simulink model "power_48pulsegtoconverter"  (R2013a)
settings: Solver=FixedStepDiscrete  SolverMode=SingleTasking  StartTime=0.0  StopTime=0.05  RelTol=1e-3
libraries: powerlib x17, powerlib_extras x1
(part 1 of 2)
Description:
  | Copyright 2008-2013 The MathWorks, Inc.
settings Model: ExtModeTrigMode=oneshot  ExtModeArmWhenConnect=off  ExtModeAutoUpdateStatusClock=off  Creator=MathWorks  LastModifiedBy=nau03113
settings DataIOCC: LimitDataPoints=off  SignalLoggingSaveFormat=ModelDataLogs  SaveOutput=off  SaveTime=off  SignalLoggingName=sigsOut
settings OptimizationCC: BlockReduction=off  BooleanDataType=off  ExpressionDepthLimit=2147483647  InitFltsAndDblsToZero=on
settings DebuggingCC: SaveWithParameterizedLinksMsg=none  CheckExecutionContextPreStartOutputMsg=on  CheckExecutionContextRuntimeOutputMsg=on  SignalResolutionControl=TryResolveAllWithWarning  SolverPrmCheckMsg=none  MultiTaskDSMMsg=warning  MultiTaskCondExecSysMsg=none  FcnCallInpInsideContextMsg=UseLocalSettings
settings HardwareCC: TargetUnknown=on
settings RTWCC: IncludeERTFirstTime=on
settings GRTTargetCC: TargetFcnLib=ansi_tfl_tmw.mat  CombineOutputUpdateFcns=off  GRTInterface=on

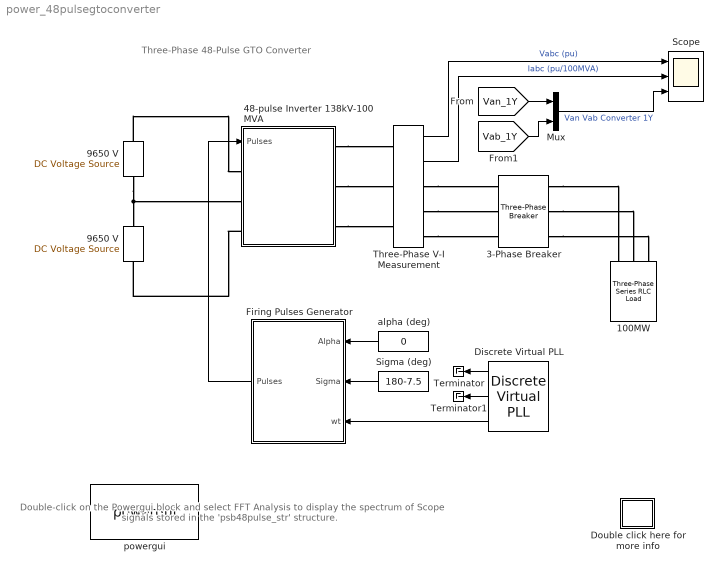
== system power_48pulsegtoconverter ==
  note: Three-Phase 48-Pulse GTO Converter
  note: Double-click on the Powergui block and
      | select FFT Analysis to display the
      | spectrum of Scope signals stored in the
      | 'psb48pulse_str' structure.
  100MW : powerlib/Elements/Three-Phase Series RLC Load  LConnTagsString=A|B|C  Configuration=Y (grounded)  NominalVoltage=138e3  NominalFrequency=60  ActivePower=100e6  InductivePower=0  CapacitivePower=0  Measurements=None  LoadType=constant Z
  3-Phase Breaker : powerlib/Elements/Three-Phase Breaker  InitialState=open  SwitchA=on  SwitchB=on  SwitchC=on  SwitchTimes=[0.025]  External=off  BreakerResistance=0.001  SnubberResistance=1e6  SnubberCapacitance=inf  Measurements=None
      settings: AttributesFormatString=\n
  48-pulse Inverter 138kV-100 MVA : Subsystem
  "9650 V " : powerlib/Electrical Sources/DC Voltage Source  Description=source block  Amplitude=9650  Measurements=None
      settings: AttributesFormatString=\n
  "9650 V  " : powerlib/Electrical Sources/DC Voltage Source  Description=source block  Amplitude=9650  Measurements=None
      settings: AttributesFormatString=\n
  Discrete Virtual PLL : powerlib_extras/Discrete  Control Blocks/Discrete Virtual PLL  Freq=60  Phase=0  Ts=5e-6
  Double click here for more info : Subsystem
      settings: OpenFcn=showdemo(bdroot(gcb))
      mask Display: disp('?')
  Firing Pulses Generator : Subsystem
  Mux : Mux  Inputs=2
  Scope : Scope  NumInputPorts=3
      settings: TimeRange=0.05  YMin=-2~-1~-20000  YMax=2~1~20000  SaveName=psb48pulse_str  SampleInput=on
  Sigma (deg) : Constant  Value=180-7.5
  Terminator : Terminator
  Terminator1 : Terminator
  Three-Phase V-I Measurement : powerlib/Measurements/Three-Phase V-I Measurement  VoltageMeasurement=phase-to-ground  SetLabelV=off  LabelV=V1  Vpu=on  VpuLL=off  CurrentMeasurement=yes  SetLabelI=off  LabelI=I1  Ipu=on  Pbase=100e6  Vbase=138e3  OutputType=Magnitude  PhasorSimulation=off  PSBequivalent=0
  alpha (deg) : Constant  Value=0  VectorParams1D=off
  powergui : powerlib/powergui  Priority=2  SimulationMode=Discrete  SolverType=Tustin  SampleTime=5e-6  frequency=60  SPID=off  DisableSnubberDevices=off  DisableRonSwitches=off  DisableVfSwitches=off  SwTol=0  Interpol=off  DisplayEquations=off  frequencyindice=1  Pbase=100e6  ErrMax=1e-4  Iterations=50  UnitsV=kV  UnitsW=MW  FunctionMessages=off  echomessages=off  HookPort=off  EnableUseOfTLC=off  x0status=blocks  RestoreLinks=warning  ResistiveCurrentMeasurement=off  Frange=logspace(0,3,50)  Ylog=off  Xlog=off  ShowGrid=off  save=off  variable=ZData  structure=psb48pulse_str  ZoomFFT=on  StartTime=0.025-1/60  cycles=1  DisplayStyle=off  fundamental=60  FreqAxis=on  MaxFrequency=4000  frequencyindicesteady=1  RmsSteady=1  display=off  Ts=0  methode=off
  wires:
  Sigma (deg)/1 -> Firing Pulses Generator/2(Sigma)
  Discrete Virtual PLL/1 -> Terminator/1
  Discrete Virtual PLL/2 -> Terminator1/1
  Firing Pulses Generator/1(Pulses) -> 48-pulse Inverter 138kV-100 MVA/1(Pulses)
  Discrete Virtual PLL/3 -> Firing Pulses Generator/3(wt)
  alpha (deg)/1 -> Firing Pulses Generator/1(Alpha)
  [Van_1Y] -> Mux/1
  [Vab_1Y] -> Mux/2
  Three-Phase V-I Measurement/1 -> Scope/1  "Vabc (pu)"
  Mux/1 -> Scope/3  "Van Vab Converter 1Y"
  Three-Phase V-I Measurement/2 -> Scope/2  "Iabc (pu/100MVA)"
  connections:
  3-Phase Breaker/RConn1 -- 100MW/LConn1
  3-Phase Breaker/RConn2 -- 100MW/LConn2
  3-Phase Breaker/RConn3 -- 100MW/LConn3
  "9650 V  "/LConn1 -- "9650 V "/RConn1 -- 48-pulse Inverter 138kV-100 MVA/LConn2
  48-pulse Inverter 138kV-100 MVA/RConn1 -- Three-Phase V-I Measurement/LConn1
  48-pulse Inverter 138kV-100 MVA/RConn2 -- Three-Phase V-I Measurement/LConn2
  48-pulse Inverter 138kV-100 MVA/RConn3 -- Three-Phase V-I Measurement/LConn3
  Three-Phase V-I Measurement/RConn1 -- 3-Phase Breaker/LConn1
  Three-Phase V-I Measurement/RConn2 -- 3-Phase Breaker/LConn2
  Three-Phase V-I Measurement/RConn3 -- 3-Phase Breaker/LConn3
  "9650 V  "/RConn1 -- 48-pulse Inverter 138kV-100 MVA/LConn1
  48-pulse Inverter 138kV-100 MVA/LConn3 -- "9650 V "/LConn1

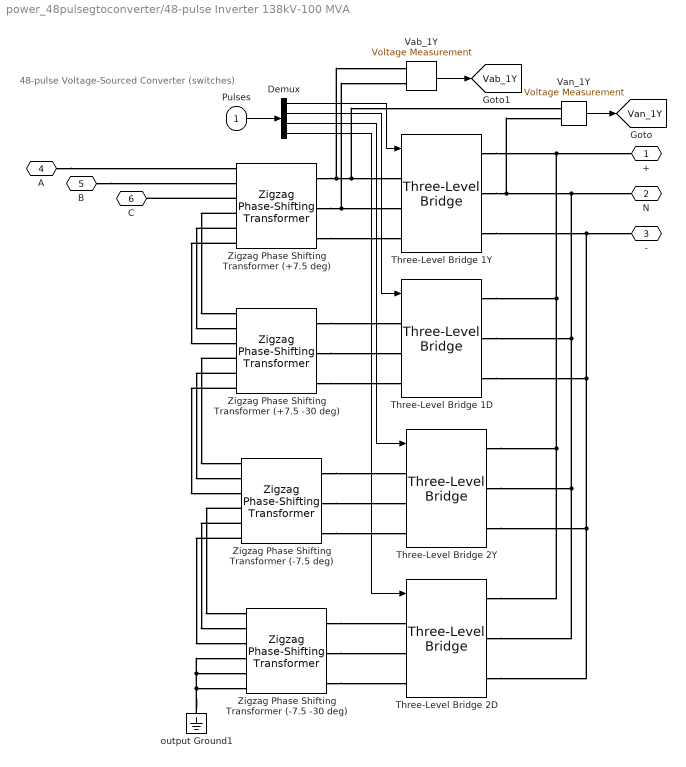
== system power_48pulsegtoconverter/48-pulse Inverter 138kV-100 MVA ==
  note: 48-pulse Voltage-Sourced Converter
      | (switches)
  Pulses : Inport  PortDimensions=48
  Demux : Demux  Outputs=[12 12 12 12]
  Three-Level Bridge 1D : powerlib/Power Electronics/Three-Level Bridge  Arms=3  SnubberResistance=1e6  SbubberCapacitance=inf  Device=Ideal Switches  Ron=1e-4  ForwardVoltages="[  0  0  ]"  Measurements=None
  Three-Level Bridge 1Y : powerlib/Power Electronics/Three-Level Bridge  Arms=3  SnubberResistance=1e6  SbubberCapacitance=inf  Device=Ideal Switches  Ron=1e-4  ForwardVoltages="[  0  0  ]"  Measurements=None
  Three-Level Bridge 2D : powerlib/Power Electronics/Three-Level Bridge  Arms=3  SnubberResistance=1e6  SbubberCapacitance=inf  Device=Ideal Switches  Ron=1e-4  ForwardVoltages="[  0  0  ]"  Measurements=None
  Three-Level Bridge 2Y : powerlib/Power Electronics/Three-Level Bridge  Arms=3  SnubberResistance=1e6  SbubberCapacitance=inf  Device=Ideal Switches  Ron=1e-4  ForwardVoltages="[  0  0  ]"  Measurements=None
  Vab_1Y : powerlib/Measurements/Voltage Measurement  Tag=PoWeRsYsTeMmEaSuReMeNt  PhasorSimulation=off  OutputType=Magnitude  PSBequivalent=0
  Van_1Y : powerlib/Measurements/Voltage Measurement  Tag=PoWeRsYsTeMmEaSuReMeNt  PhasorSimulation=off  OutputType=Magnitude  PSBequivalent=0
  Zigzag Phase Shifting Transformer (+7.5 -30 deg) : powerlib/Elements/Zigzag Phase-Shifting Transformer  SecondaryConnection=Delta D1(-30 deg.)  UNITS=pu  NominalPower=[ 25e6 60]  PrimaryVoltage=138e3/4  SecondaryVoltage="[ 15e3  +7.5]"  Winding1=[ 0.00125 0.05 ]  Winding2=[ 0.00125 0.05 ]  Winding3=[ 0.00125 0.05 ]  SetSaturation=off  RmLm=[ 500 500 ]  Rm=500  Saturation="[ 0,0  ;  0.005,1.2  ;  1.0,1.4 ]"  SetInitialFlux=off  Measurements=Fluxes and magnetization currents (Imag)  InitialFluxes=[0,0,0]  MoreParameters=off  BreakLoop=off  DataType=off
      settings: AttributesFormatString=\n
  Zigzag Phase Shifting Transformer (+7.5 deg) : powerlib/Elements/Zigzag Phase-Shifting Transformer  SecondaryConnection=Y  UNITS=pu  NominalPower=[ 25e6 60]  PrimaryVoltage=138e3/4  SecondaryVoltage="[ 15e3  +7.5]"  Winding1=[ 0.00125 0.05 ]  Winding2=[ 0.00125 0.05 ]  Winding3=[ 0.00125 0.05 ]  SetSaturation=off  RmLm=[ 500 500 ]  Rm=500  Saturation="[ 0,0  ;  0.005,1.2  ;  1.0,1.4 ]"  SetInitialFlux=off  Measurements=Fluxes and excitation currents (Imag + IRm)  InitialFluxes=[0,0,0]  MoreParameters=off  BreakLoop=off  DataType=off
      settings: AttributesFormatString=\n
  Zigzag Phase Shifting Transformer (-7.5 -30 deg) : powerlib/Elements/Zigzag Phase-Shifting Transformer  SecondaryConnection=Delta D1(-30 deg.)  UNITS=pu  NominalPower=[ 25e6 60]  PrimaryVoltage=138e3/4  SecondaryVoltage="[ 15e3  -7.5]"  Winding1=[ 0.00125 0.05 ]  Winding2=[ 0.00125 0.05 ]  Winding3=[ 0.00125 0.05 ]  SetSaturation=off  RmLm=[ 500 500 ]  Rm=500  Saturation="[ 0,0  ;  0.005,1.2  ;  1.0,1.4 ]"  SetInitialFlux=off  Measurements=None  InitialFluxes=[0,0,0]  MoreParameters=off  BreakLoop=off  DataType=off
      settings: AttributesFormatString=\n
  Zigzag Phase Shifting Transformer (-7.5 deg) : powerlib/Elements/Zigzag Phase-Shifting Transformer  SecondaryConnection=Y  UNITS=pu  NominalPower=[ 25e6 60]  PrimaryVoltage=138e3/4  SecondaryVoltage="[ 15e3  -7.5]"  Winding1=[ 0.00125 0.05 ]  Winding2=[ 0.00125 0.05 ]  Winding3=[ 0.00125 0.05 ]  SetSaturation=off  RmLm=[ 500 500 ]  Rm=500  Saturation="[ 0,0  ;  0.005,1.2  ;  1.0,1.4 ]"  SetInitialFlux=off  Measurements=None  InitialFluxes=[0,0,0]  MoreParameters=off  BreakLoop=off  DataType=off
      settings: AttributesFormatString=\n
  output Ground1 : powerlib/Elements/Ground  LConnTagsString=a
  + : PMIOPort  Port=1  Side=Left
  N : PMIOPort  Port=2  Side=Left
  - : PMIOPort  Port=3  Side=Left
  A : PMIOPort  Port=4  Side=Right
  B : PMIOPort  Port=5  Side=Right
  C : PMIOPort  Port=6  Side=Right
  tag scope: Vab_1Y=global, Van_1Y=global
  wires:
  Pulses/1 -> Demux/1
  Van_1Y/1 -> [Van_1Y]
  Vab_1Y/1 -> [Vab_1Y]
  Demux/1 -> Three-Level Bridge 1Y/1
  Demux/2 -> Three-Level Bridge 1D/1
  Demux/3 -> Three-Level Bridge 2Y/1
  Demux/4 -> Three-Level Bridge 2D/1
  connections:
  output Ground1/LConn1 -- Zigzag Phase Shifting Transformer (-7.5 -30 deg)/LConn5 -- Zigzag Phase Shifting Transformer (-7.5 -30 deg)/LConn4 -- Zigzag Phase Shifting Transformer (-7.5 -30 deg)/LConn6
  Zigzag Phase Shifting Transformer (+7.5 -30 deg)/RConn1 -- Three-Level Bridge 1D/LConn1
  Zigzag Phase Shifting Transformer (+7.5 -30 deg)/RConn2 -- Three-Level Bridge 1D/LConn2
  Zigzag Phase Shifting Transformer (+7.5 -30 deg)/RConn3 -- Three-Level Bridge 1D/LConn3
  Zigzag Phase Shifting Transformer (-7.5 deg)/RConn1 -- Three-Level Bridge 2Y/LConn1
  Zigzag Phase Shifting Transformer (-7.5 deg)/RConn2 -- Three-Level Bridge 2Y/LConn2
  Zigzag Phase Shifting Transformer (-7.5 deg)/RConn3 -- Three-Level Bridge 2Y/LConn3
  Zigzag Phase Shifting Transformer (-7.5 -30 deg)/RConn1 -- Three-Level Bridge 2D/LConn1
  Zigzag Phase Shifting Transformer (-7.5 -30 deg)/RConn2 -- Three-Level Bridge 2D/LConn2
  Zigzag Phase Shifting Transformer (-7.5 -30 deg)/RConn3 -- Three-Level Bridge 2D/LConn3
  A/RConn1 -- Zigzag Phase Shifting Transformer (+7.5 deg)/LConn1
  B/RConn1 -- Zigzag Phase Shifting Transformer (+7.5 deg)/LConn2
  Zigzag Phase Shifting Transformer (+7.5 deg)/LConn3 -- C/RConn1
  Zigzag Phase Shifting Transformer (+7.5 deg)/RConn2 -- Three-Level Bridge 1Y/LConn2 -- Vab_1Y/LConn2
  Zigzag Phase Shifting Transformer (+7.5 deg)/RConn1 -- Vab_1Y/LConn1 -- Three-Level Bridge 1Y/LConn1 -- Van_1Y/LConn1
  Zigzag Phase Shifting Transformer (+7.5 deg)/RConn3 -- Three-Level Bridge 1Y/LConn3
  Zigzag Phase Shifting Transformer (+7.5 deg)/LConn4 -- Zigzag Phase Shifting Transformer (+7.5 -30 deg)/LConn1
  Zigzag Phase Shifting Transformer (+7.5 deg)/LConn5 -- Zigzag Phase Shifting Transformer (+7.5 -30 deg)/LConn2
  Zigzag Phase Shifting Transformer (+7.5 deg)/LConn6 -- Zigzag Phase Shifting Transformer (+7.5 -30 deg)/LConn3
  Zigzag Phase Shifting Transformer (+7.5 -30 deg)/LConn4 -- Zigzag Phase Shifting Transformer (-7.5 deg)/LConn1
  Zigzag Phase Shifting Transformer (+7.5 -30 deg)/LConn5 -- Zigzag Phase Shifting Transformer (-7.5 deg)/LConn2
  Zigzag Phase Shifting Transformer (+7.5 -30 deg)/LConn6 -- Zigzag Phase Shifting Transformer (-7.5 deg)/LConn3
  Zigzag Phase Shifting Transformer (-7.5 deg)/LConn5 -- Zigzag Phase Shifting Transformer (-7.5 -30 deg)/LConn2
  Three-Level Bridge 1Y/RConn2 -- N/RConn1 -- Three-Level Bridge 1D/RConn2 -- Three-Level Bridge 2D/RConn2 -- Three-Level Bridge 2Y/RConn2 -- Van_1Y/LConn2
  Three-Level Bridge 2D/RConn1 -- Three-Level Bridge 2Y/RConn1 -- Three-Level Bridge 1Y/RConn1 -- +/RConn1 -- Three-Level Bridge 1D/RConn1
  Three-Level Bridge 2D/RConn3 -- Three-Level Bridge 2Y/RConn3 -- Three-Level Bridge 1Y/RConn3 -- -/RConn1 -- Three-Level Bridge 1D/RConn3
  Zigzag Phase Shifting Transformer (-7.5 deg)/LConn4 -- Zigzag Phase Shifting Transformer (-7.5 -30 deg)/LConn1
  Zigzag Phase Shifting Transformer (-7.5 deg)/LConn6 -- Zigzag Phase Shifting Transformer (-7.5 -30 deg)/LConn3

== system power_48pulsegtoconverter/Double click here for more info ==

== system power_48pulsegtoconverter/Firing Pulses Generator ==
  Alpha : Inport  PortDimensions=1
  Sigma : Inport  Port=2  PortDimensions=1
  wt : Inport  Port=3  PortDimensions=1
  Bridge 1D : Subsystem
  "Bridge 1Y " : Subsystem
  Bridge 2D : Subsystem
  Bridge 2Y : Subsystem
  Constant : Constant  Value=[0 -30 -15 -45]*pi/180
  Deg->Rad : Gain  Gain=pi/180  SaturateOnIntegerOverflow=on  OutDataTypeStr=Inherit: Same as input  ParamDataTypeStr=Inherit: Same as input
  "Deg->Rad " : Gain  Gain=pi/180  SaturateOnIntegerOverflow=on  OutDataTypeStr=Inherit: Same as input  ParamDataTypeStr=Inherit: Same as input
  Demux : Demux
  Mux : Mux  Inputs=[12 12 12 12]
  Sum : Sum  SaturateOnIntegerOverflow=on  InputSameDT=on  OutDataTypeStr=Inherit: Same as first input
  Pulses : Outport
  wires:
  Alpha/1 -> Deg->Rad/1
  Constant/1 -> Sum/2
  "Bridge 1Y "/1(Pulses) -> Mux/1
  Mux/1 -> Pulses/1
  Demux/1 -> "Bridge 1Y "/1(wt)
  Sigma/1 -> "Deg->Rad "/1
  Demux/2 -> Bridge 1D/1(wt)
  Demux/3 -> Bridge 2Y/1(wt)
  Demux/4 -> Bridge 2D/1(wt)
  Deg->Rad/1 -> "Bridge 1Y "/2(Alpha), Bridge 2Y/2(Alpha), Bridge 2D/2(Alpha), Bridge 1D/2(Alpha)
  "Deg->Rad "/1 -> "Bridge 1Y "/3(Sigma), Bridge 1D/3(Sigma), Bridge 2Y/3(Sigma), Bridge 2D/3(Sigma)
  Bridge 1D/1(Pulses) -> Mux/2
  Bridge 2Y/1(Pulses) -> Mux/3
  Bridge 2D/1(Pulses) -> Mux/4
  wt/1 -> Sum/1
  Sum/1 -> Demux/1

== system power_48pulsegtoconverter/Firing Pulses Generator/Bridge 1D ==
  wt : Inport  PortDimensions=1
  Alpha : Inport  Port=2  PortDimensions=1
  Sigma : Inport  Port=3  PortDimensions=1
  Constant : Constant  Value=-2*pi/3
  Constant1 : Constant  Value=2*pi/3
  Mux1 : Mux  Inputs=[4 4 4]
  Phase A : Subsystem
  Phase B : Subsystem
  Phase C : Subsystem
  Sum : Sum  SaturateOnIntegerOverflow=on  InputSameDT=on  OutDataTypeStr=Inherit: Same as first input
  Sum1 : Sum  SaturateOnIntegerOverflow=on  InputSameDT=on  OutDataTypeStr=Inherit: Same as first input
  Sum2 : Sum  SaturateOnIntegerOverflow=on  InputSameDT=on  OutDataTypeStr=Inherit: Same as first input
  Pulses : Outport
  wires:
  Constant1/1 -> Sum1/2
  Sigma/1 -> Phase A/2(sigma), Phase C/2(sigma), Phase B/2(sigma)
  Alpha/1 -> Sum2/2
  wt/1 -> Sum2/1
  Sum2/1 -> Phase A/1(wt), Sum/1, Sum1/1
  Mux1/1 -> Pulses/1
  Phase A/1(Pulses) -> Mux1/1
  Constant/1 -> Sum/2
  Sum/1 -> Phase B/1(wt)
  Sum1/1 -> Phase C/1(wt)
  Phase B/1(Pulses) -> Mux1/2
  Phase C/1(Pulses) -> Mux1/3

== system power_48pulsegtoconverter/Firing Pulses Generator/Bridge 1Y  ==
  wt : Inport  PortDimensions=1
  Alpha : Inport  Port=2  PortDimensions=1
  Sigma : Inport  Port=3  PortDimensions=1
  Constant : Constant  Value=-2*pi/3
  Constant1 : Constant  Value=2*pi/3
  Mux1 : Mux  Inputs=[4 4 4]
  Phase A : Subsystem
  Phase B : Subsystem
  Phase C : Subsystem
  Sum : Sum  SaturateOnIntegerOverflow=on  InputSameDT=on  OutDataTypeStr=Inherit: Same as first input
  Sum1 : Sum  SaturateOnIntegerOverflow=on  InputSameDT=on  OutDataTypeStr=Inherit: Same as first input
  Sum2 : Sum  SaturateOnIntegerOverflow=on  InputSameDT=on  OutDataTypeStr=Inherit: Same as first input
  Pulses : Outport
  wires:
  Phase C/1(Pulses) -> Mux1/3
  Phase B/1(Pulses) -> Mux1/2
  Sum1/1 -> Phase C/1(wt)
  Sum/1 -> Phase B/1(wt)
  Constant/1 -> Sum/2
  Phase A/1(Pulses) -> Mux1/1
  Mux1/1 -> Pulses/1
  Sum2/1 -> Sum1/1, Sum/1, Phase A/1(wt)
  wt/1 -> Sum2/1
  Alpha/1 -> Sum2/2
  Sigma/1 -> Phase B/2(sigma), Phase C/2(sigma), Phase A/2(sigma)
  Constant1/1 -> Sum1/2

== system power_48pulsegtoconverter/Firing Pulses Generator/Bridge 2D ==
  wt : Inport  PortDimensions=1
  Alpha : Inport  Port=2  PortDimensions=1
  Sigma : Inport  Port=3  PortDimensions=1
  Constant : Constant  Value=-2*pi/3
  Constant1 : Constant  Value=2*pi/3
  Mux1 : Mux  Inputs=[4 4 4]
  Phase A : Subsystem
  Phase B : Subsystem
  Phase C : Subsystem
  Sum : Sum  SaturateOnIntegerOverflow=on  InputSameDT=on  OutDataTypeStr=Inherit: Same as first input
  Sum1 : Sum  SaturateOnIntegerOverflow=on  InputSameDT=on  OutDataTypeStr=Inherit: Same as first input
  Sum2 : Sum  SaturateOnIntegerOverflow=on  InputSameDT=on  OutDataTypeStr=Inherit: Same as first input
  Pulses : Outport
  wires:
  Constant1/1 -> Sum1/2
  Sigma/1 -> Phase A/2(sigma), Phase C/2(sigma), Phase B/2(sigma)
  Alpha/1 -> Sum2/2
  wt/1 -> Sum2/1
  Sum2/1 -> Phase A/1(wt), Sum/1, Sum1/1
  Mux1/1 -> Pulses/1
  Phase A/1(Pulses) -> Mux1/1
  Constant/1 -> Sum/2
  Sum/1 -> Phase B/1(wt)
  Sum1/1 -> Phase C/1(wt)
  Phase B/1(Pulses) -> Mux1/2
  Phase C/1(Pulses) -> Mux1/3

== system power_48pulsegtoconverter/Firing Pulses Generator/Bridge 2Y ==
  wt : Inport  PortDimensions=1
  Alpha : Inport  Port=2  PortDimensions=1
  Sigma : Inport  Port=3  PortDimensions=1
  Constant : Constant  Value=-2*pi/3
  Constant1 : Constant  Value=2*pi/3
  Mux1 : Mux  Inputs=[4 4 4]
  Phase A : Subsystem
  Phase B : Subsystem
  Phase C : Subsystem
  Sum : Sum  SaturateOnIntegerOverflow=on  InputSameDT=on  OutDataTypeStr=Inherit: Same as first input
  Sum1 : Sum  SaturateOnIntegerOverflow=on  InputSameDT=on  OutDataTypeStr=Inherit: Same as first input
  Sum2 : Sum  SaturateOnIntegerOverflow=on  InputSameDT=on  OutDataTypeStr=Inherit: Same as first input
  Pulses : Outport
  wires:
  Phase C/1(Pulses) -> Mux1/3
  Phase B/1(Pulses) -> Mux1/2
  Sum1/1 -> Phase C/1(wt)
  Sum/1 -> Phase B/1(wt)
  Constant/1 -> Sum/2
  Phase A/1(Pulses) -> Mux1/1
  Mux1/1 -> Pulses/1
  Sum2/1 -> Sum1/1, Sum/1, Phase A/1(wt)
  wt/1 -> Sum2/1
  Alpha/1 -> Sum2/2
  Sigma/1 -> Phase B/2(sigma), Phase C/2(sigma), Phase A/2(sigma)
  Constant1/1 -> Sum1/2

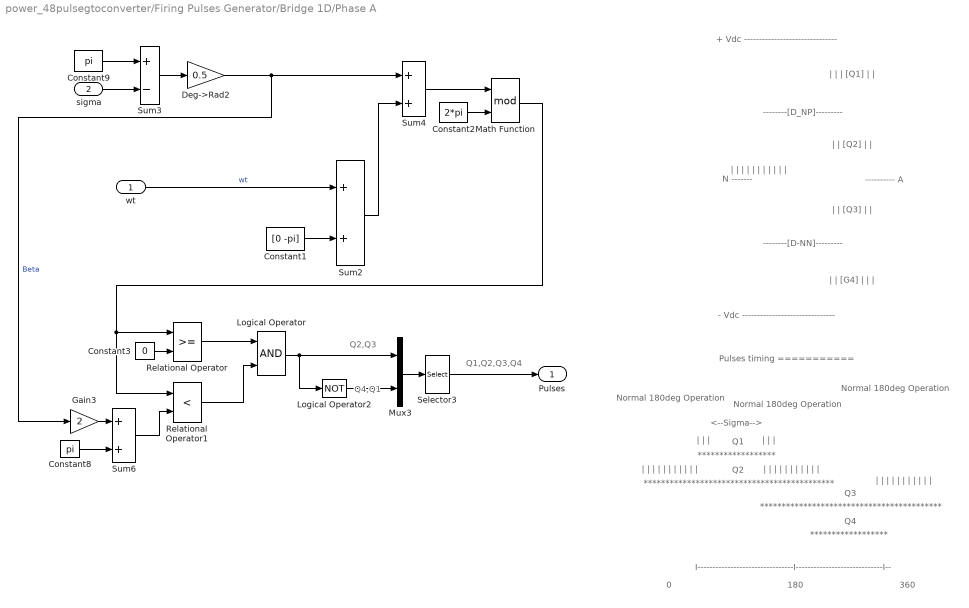
== system power_48pulsegtoconverter/Firing Pulses Generator/Bridge 1D/Phase A ==
  note: <--Sigma-->
  note: |
      | |
      | |
  note: |
      | |
      | |
  note: Q4
  note: Q3
  note: Q2
  note: Q1
  note: ******************************************
  note: ********************************************
  note: ******************
  note: ******************
  note: 360
  note: 180
  note: 0
  note: I--------------------------------I-----------------------------I--
  note: Normal 180deg
      | Operation
  note: Normal 180deg
      | Operation
  note: Normal 180deg
      | Operation
  note: Pulses timing
      | ===========
  note: |
      | |
      | |
      | |
      | |
      | |
      | |
      | |
      | |
      | |
      | |
  note: |
      | |
      | |
      | |
      | |
      | |
      | |
      | |
      | |
      | |
      | |
  note: |
      | |
      | |
      | |
      | |
      | |
      | |
      | |
      | |
      | |
      | |
  note: Q1,Q2,Q3,Q4
  note: Q2,Q3
  note: Q4,Q1
  note: + Vdc -------------------------------
  note: - Vdc -------------------------------
  note: N -------
  note: |
      | |
      | |
      | |
      | |
      | |
      | |
      | |
      | |
      | |
      | |
  note: ---------- A
  note: --------[D-NN]---------
  note: --------[D_NP]---------
  note: |
      | |
      | [G4]
      | |
      | |
      | |
  note: |
      | |
      | [Q3]
      | |
      | |
  note: |
      | |
      | [Q2]
      | |
      | |
  note: |
      | |
      | |
      | [Q1]
      | |
      | |
  wt : Inport  PortDimensions=1
  sigma : Inport  Port=2  PortDimensions=1
  Constant1 : Constant  Value=[0 -pi]
  Constant2 : Constant  Value=2*pi
  Constant3 : Constant  Value=0
  Constant8 : Constant  Value=pi
  Constant9 : Constant  Value=pi
  Deg->Rad2 : Gain  Gain=0.5  SaturateOnIntegerOverflow=on  OutDataTypeStr=Inherit: Same as input  ParamDataTypeStr=Inherit: Same as input
  Gain3 : Gain  Gain=2  SaturateOnIntegerOverflow=on  OutDataTypeStr=Inherit: Same as input  ParamDataTypeStr=Inherit: Same as input
  Logical Operator : Logic
  Logical Operator2 : Logic  Operator=NOT
  Math Function : Math  Operator=mod  SaturateOnIntegerOverflow=on
  Mux3 : Mux  Inputs=[2 2]
  Relational Operator : RelationalOperator  ZeroCross=off  InputSameDT=on
  Relational Operator1 : RelationalOperator  Operator=<  ZeroCross=off  InputSameDT=on
  Selector3 : Selector  InputPortWidth=4  IndexOptions=Index vector (dialog)  Indices=[4 1 2 3]  OutputSizes=1
  Sum2 : Sum  SaturateOnIntegerOverflow=on  InputSameDT=on  OutDataTypeStr=Inherit: Same as first input
  Sum3 : Sum  Inputs=+-  SaturateOnIntegerOverflow=on  InputSameDT=on  OutDataTypeStr=Inherit: Same as first input
  Sum4 : Sum  SaturateOnIntegerOverflow=on  InputSameDT=on  OutDataTypeStr=Inherit: Same as first input
  Sum6 : Sum  SaturateOnIntegerOverflow=on  InputSameDT=on  OutDataTypeStr=Inherit: Same as first input
  Pulses : Outport
  wires:
  Constant2/1 -> Math Function/2
  wt/1 -> Sum2/1  "wt"
  Math Function/1 -> Relational Operator/1, Relational Operator1/1
  Gain3/1 -> Sum6/1
  Selector3/1 -> Pulses/1
  Mux3/1 -> Selector3/1
  Logical Operator2/1 -> Mux3/2
  Logical Operator/1 -> Mux3/1, Logical Operator2/1
  Sum4/1 -> Math Function/1
  Sum2/1 -> Sum4/2
  Sum6/1 -> Relational Operator1/2
  Constant8/1 -> Sum6/2
  Deg->Rad2/1 -> Gain3/1, Sum4/1  "Beta"
  Sum3/1 -> Deg->Rad2/1
  sigma/1 -> Sum3/2
  Constant9/1 -> Sum3/1
  Relational Operator1/1 -> Logical Operator/2
  Relational Operator/1 -> Logical Operator/1
  Constant3/1 -> Relational Operator/2
  Constant1/1 -> Sum2/2

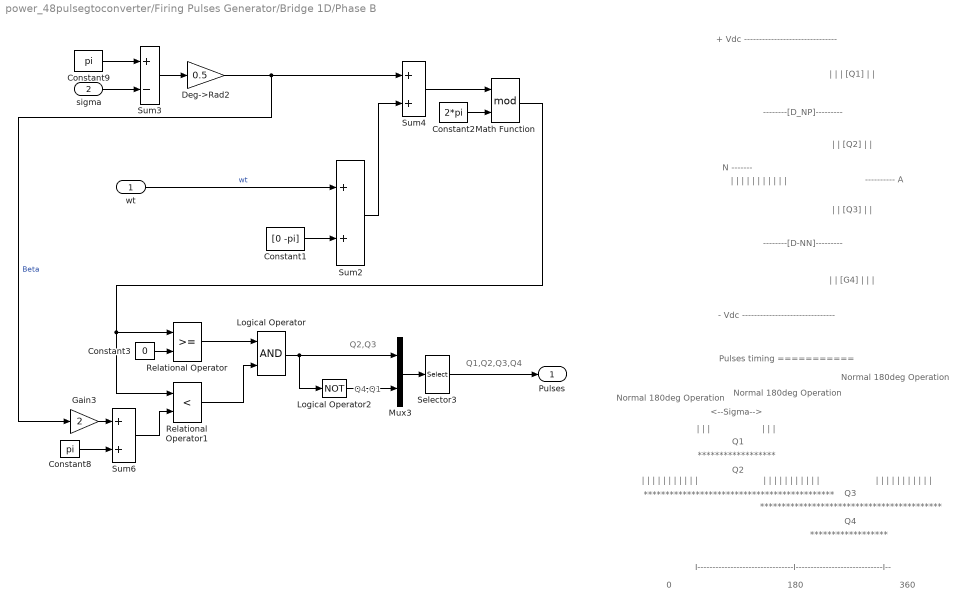
== system power_48pulsegtoconverter/Firing Pulses Generator/Bridge 1D/Phase B ==
  note: |
      | |
      | |
      | [Q1]
      | |
      | |
  note: |
      | |
      | [Q2]
      | |
      | |
  note: |
      | |
      | [Q3]
      | |
      | |
  note: |
      | |
      | [G4]
      | |
      | |
      | |
  note: --------[D_NP]---------
  note: --------[D-NN]---------
  note: ---------- A
  note: |
      | |
      | |
      | |
      | |
      | |
      | |
      | |
      | |
      | |
      | |
  note: N -------
  note: - Vdc -------------------------------
  note: + Vdc -------------------------------
  note: Q4,Q1
  note: Q2,Q3
  note: Q1,Q2,Q3,Q4
  note: |
      | |
      | |
      | |
      | |
      | |
      | |
      | |
      | |
      | |
      | |
  note: |
      | |
      | |
      | |
      | |
      | |
      | |
      | |
      | |
      | |
      | |
  note: |
      | |
      | |
      | |
      | |
      | |
      | |
      | |
      | |
      | |
      | |
  note: Pulses timing
      | ===========
  note: Normal 180deg
      | Operation
  note: Normal 180deg
      | Operation
  note: Normal 180deg
      | Operation
  note: I--------------------------------I-----------------------------I--
  note: 0
  note: 180
  note: 360
  note: ******************
  note: ******************
  note: ********************************************
  note: ******************************************
  note: Q1
  note: Q2
  note: Q3
  note: Q4
  note: |
      | |
      | |
  note: |
      | |
      | |
  note: <--Sigma-->
  wt : Inport  PortDimensions=1
  sigma : Inport  Port=2  PortDimensions=1
  Constant1 : Constant  Value=[0 -pi]
  Constant2 : Constant  Value=2*pi
  Constant3 : Constant  Value=0
  Constant8 : Constant  Value=pi
  Constant9 : Constant  Value=pi
  Deg->Rad2 : Gain  Gain=0.5  SaturateOnIntegerOverflow=on  OutDataTypeStr=Inherit: Same as input  ParamDataTypeStr=Inherit: Same as input
  Gain3 : Gain  Gain=2  SaturateOnIntegerOverflow=on  OutDataTypeStr=Inherit: Same as input  ParamDataTypeStr=Inherit: Same as input
  Logical Operator : Logic
  Logical Operator2 : Logic  Operator=NOT
  Math Function : Math  Operator=mod  SaturateOnIntegerOverflow=on
  Mux3 : Mux  Inputs=[2 2]
  Relational Operator : RelationalOperator  ZeroCross=off  InputSameDT=on
  Relational Operator1 : RelationalOperator  Operator=<  ZeroCross=off  InputSameDT=on
  Selector3 : Selector  InputPortWidth=4  IndexOptions=Index vector (dialog)  Indices=[4 1 2 3]  OutputSizes=1
  Sum2 : Sum  SaturateOnIntegerOverflow=on  InputSameDT=on  OutDataTypeStr=Inherit: Same as first input
  Sum3 : Sum  Inputs=+-  SaturateOnIntegerOverflow=on  InputSameDT=on  OutDataTypeStr=Inherit: Same as first input
  Sum4 : Sum  SaturateOnIntegerOverflow=on  InputSameDT=on  OutDataTypeStr=Inherit: Same as first input
  Sum6 : Sum  SaturateOnIntegerOverflow=on  InputSameDT=on  OutDataTypeStr=Inherit: Same as first input
  Pulses : Outport
  wires:
  Constant1/1 -> Sum2/2
  Constant3/1 -> Relational Operator/2
  Relational Operator/1 -> Logical Operator/1
  Relational Operator1/1 -> Logical Operator/2
  Constant9/1 -> Sum3/1
  sigma/1 -> Sum3/2
  Sum3/1 -> Deg->Rad2/1
  Deg->Rad2/1 -> Sum4/1, Gain3/1  "Beta"
  Constant8/1 -> Sum6/2
  Sum6/1 -> Relational Operator1/2
  Sum2/1 -> Sum4/2
  Sum4/1 -> Math Function/1
  Logical Operator/1 -> Logical Operator2/1, Mux3/1
  Logical Operator2/1 -> Mux3/2
  Mux3/1 -> Selector3/1
  Selector3/1 -> Pulses/1
  Gain3/1 -> Sum6/1
  Math Function/1 -> Relational Operator1/1, Relational Operator/1
  wt/1 -> Sum2/1  "wt"
  Constant2/1 -> Math Function/2

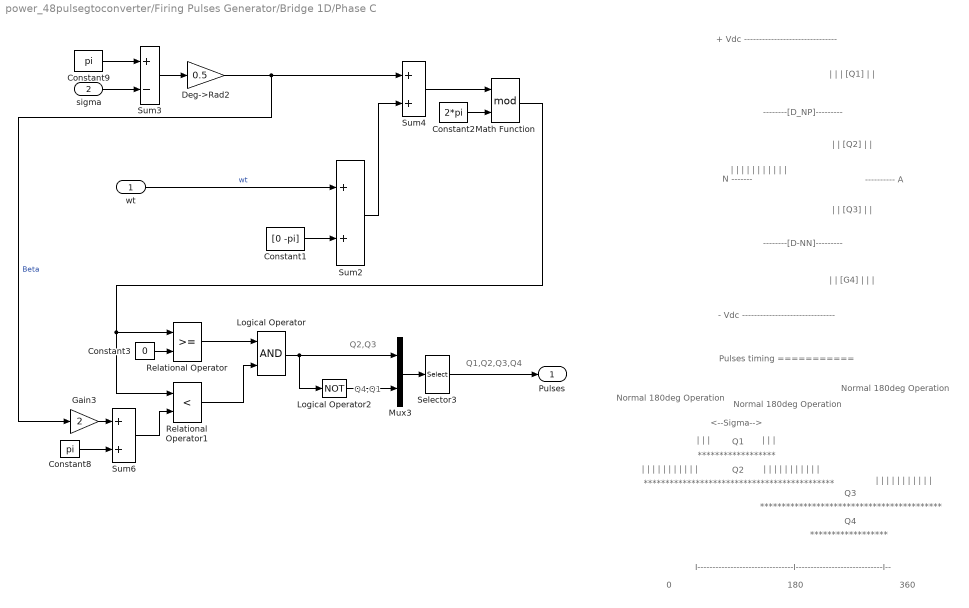
== system power_48pulsegtoconverter/Firing Pulses Generator/Bridge 1D/Phase C ==
  note: <--Sigma-->
  note: |
      | |
      | |
  note: |
      | |
      | |
  note: Q4
  note: Q3
  note: Q2
  note: Q1
  note: ******************************************
  note: ********************************************
  note: ******************
  note: ******************
  note: 360
  note: 180
  note: 0
  note: I--------------------------------I-----------------------------I--
  note: Normal 180deg
      | Operation
  note: Normal 180deg
      | Operation
  note: Normal 180deg
      | Operation
  note: Pulses timing
      | ===========
  note: |
      | |
      | |
      | |
      | |
      | |
      | |
      | |
      | |
      | |
      | |
  note: |
      | |
      | |
      | |
      | |
      | |
      | |
      | |
      | |
      | |
      | |
  note: |
      | |
      | |
      | |
      | |
      | |
      | |
      | |
      | |
      | |
      | |
  note: Q1,Q2,Q3,Q4
  note: Q2,Q3
  note: Q4,Q1
  note: + Vdc -------------------------------
  note: - Vdc -------------------------------
  note: N -------
  note: |
      | |
      | |
      | |
      | |
      | |
      | |
      | |
      | |
      | |
      | |
  note: ---------- A
  note: --------[D-NN]---------
  note: --------[D_NP]---------
  note: |
      | |
      | [G4]
      | |
      | |
      | |
  note: |
      | |
      | [Q3]
      | |
      | |
  note: |
      | |
      | [Q2]
      | |
      | |
  note: |
      | |
      | |
      | [Q1]
      | |
      | |
  wt : Inport  PortDimensions=1
  sigma : Inport  Port=2  PortDimensions=1
  Constant1 : Constant  Value=[0 -pi]
  Constant2 : Constant  Value=2*pi
  Constant3 : Constant  Value=0
  Constant8 : Constant  Value=pi
  Constant9 : Constant  Value=pi
  Deg->Rad2 : Gain  Gain=0.5  SaturateOnIntegerOverflow=on  OutDataTypeStr=Inherit: Same as input  ParamDataTypeStr=Inherit: Same as input
  Gain3 : Gain  Gain=2  SaturateOnIntegerOverflow=on  OutDataTypeStr=Inherit: Same as input  ParamDataTypeStr=Inherit: Same as input
  Logical Operator : Logic
  Logical Operator2 : Logic  Operator=NOT
  Math Function : Math  Operator=mod  SaturateOnIntegerOverflow=on
  Mux3 : Mux  Inputs=[2 2]
  Relational Operator : RelationalOperator  ZeroCross=off  InputSameDT=on
  Relational Operator1 : RelationalOperator  Operator=<  ZeroCross=off  InputSameDT=on
  Selector3 : Selector  InputPortWidth=4  IndexOptions=Index vector (dialog)  Indices=[4 1 2 3]  OutputSizes=1
  Sum2 : Sum  SaturateOnIntegerOverflow=on  InputSameDT=on  OutDataTypeStr=Inherit: Same as first input
  Sum3 : Sum  Inputs=+-  SaturateOnIntegerOverflow=on  InputSameDT=on  OutDataTypeStr=Inherit: Same as first input
  Sum4 : Sum  SaturateOnIntegerOverflow=on  InputSameDT=on  OutDataTypeStr=Inherit: Same as first input
  Sum6 : Sum  SaturateOnIntegerOverflow=on  InputSameDT=on  OutDataTypeStr=Inherit: Same as first input
  Pulses : Outport
  wires:
  Constant2/1 -> Math Function/2
  wt/1 -> Sum2/1  "wt"
  Math Function/1 -> Relational Operator/1, Relational Operator1/1
  Gain3/1 -> Sum6/1
  Selector3/1 -> Pulses/1
  Mux3/1 -> Selector3/1
  Logical Operator2/1 -> Mux3/2
  Logical Operator/1 -> Mux3/1, Logical Operator2/1
  Sum4/1 -> Math Function/1
  Sum2/1 -> Sum4/2
  Sum6/1 -> Relational Operator1/2
  Constant8/1 -> Sum6/2
  Deg->Rad2/1 -> Gain3/1, Sum4/1  "Beta"
  Sum3/1 -> Deg->Rad2/1
  sigma/1 -> Sum3/2
  Constant9/1 -> Sum3/1
  Relational Operator1/1 -> Logical Operator/2
  Relational Operator/1 -> Logical Operator/1
  Constant3/1 -> Relational Operator/2
  Constant1/1 -> Sum2/2

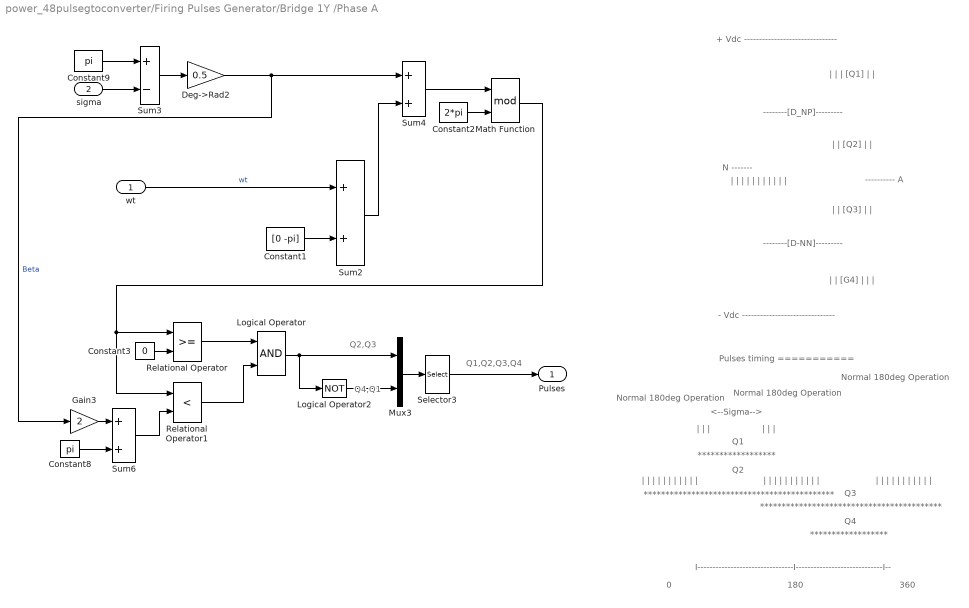
== system power_48pulsegtoconverter/Firing Pulses Generator/Bridge 1Y /Phase A ==
  note: |
      | |
      | |
      | [Q1]
      | |
      | |
  note: |
      | |
      | [Q2]
      | |
      | |
  note: |
      | |
      | [Q3]
      | |
      | |
  note: |
      | |
      | [G4]
      | |
      | |
      | |
  note: --------[D_NP]---------
  note: --------[D-NN]---------
  note: ---------- A
  note: |
      | |
      | |
      | |
      | |
      | |
      | |
      | |
      | |
      | |
      | |
  note: N -------
  note: - Vdc -------------------------------
  note: + Vdc -------------------------------
  note: Q4,Q1
  note: Q2,Q3
  note: Q1,Q2,Q3,Q4
  note: |
      | |
      | |
      | |
      | |
      | |
      | |
      | |
      | |
      | |
      | |
  note: |
      | |
      | |
      | |
      | |
      | |
      | |
      | |
      | |
      | |
      | |
  note: |
      | |
      | |
      | |
      | |
      | |
      | |
      | |
      | |
      | |
      | |
  note: Pulses timing
      | ===========
  note: Normal 180deg
      | Operation
  note: Normal 180deg
      | Operation
  note: Normal 180deg
      | Operation
  note: I--------------------------------I-----------------------------I--
  note: 0
  note: 180
  note: 360
  note: ******************
  note: ******************
  note: ********************************************
  note: ******************************************
  note: Q1
  note: Q2
  note: Q3
  note: Q4
  note: |
      | |
      | |
  note: |
      | |
      | |
  note: <--Sigma-->
  wt : Inport  PortDimensions=1
  sigma : Inport  Port=2  PortDimensions=1
  Constant1 : Constant  Value=[0 -pi]
  Constant2 : Constant  Value=2*pi
  Constant3 : Constant  Value=0
  Constant8 : Constant  Value=pi
  Constant9 : Constant  Value=pi
  Deg->Rad2 : Gain  Gain=0.5  SaturateOnIntegerOverflow=on  OutDataTypeStr=Inherit: Same as input  ParamDataTypeStr=Inherit: Same as input
  Gain3 : Gain  Gain=2  SaturateOnIntegerOverflow=on  OutDataTypeStr=Inherit: Same as input  ParamDataTypeStr=Inherit: Same as input
  Logical Operator : Logic
  Logical Operator2 : Logic  Operator=NOT
  Math Function : Math  Operator=mod  SaturateOnIntegerOverflow=on
  Mux3 : Mux  Inputs=[2 2]
  Relational Operator : RelationalOperator  ZeroCross=off  InputSameDT=on
  Relational Operator1 : RelationalOperator  Operator=<  ZeroCross=off  InputSameDT=on
  Selector3 : Selector  InputPortWidth=4  IndexOptions=Index vector (dialog)  Indices=[4 1 2 3]  OutputSizes=1
  Sum2 : Sum  SaturateOnIntegerOverflow=on  InputSameDT=on  OutDataTypeStr=Inherit: Same as first input
  Sum3 : Sum  Inputs=+-  SaturateOnIntegerOverflow=on  InputSameDT=on  OutDataTypeStr=Inherit: Same as first input
  Sum4 : Sum  SaturateOnIntegerOverflow=on  InputSameDT=on  OutDataTypeStr=Inherit: Same as first input
  Sum6 : Sum  SaturateOnIntegerOverflow=on  InputSameDT=on  OutDataTypeStr=Inherit: Same as first input
  Pulses : Outport
  wires:
  Constant1/1 -> Sum2/2
  Constant3/1 -> Relational Operator/2
  Relational Operator/1 -> Logical Operator/1
  Relational Operator1/1 -> Logical Operator/2
  Constant9/1 -> Sum3/1
  sigma/1 -> Sum3/2
  Sum3/1 -> Deg->Rad2/1
  Deg->Rad2/1 -> Sum4/1, Gain3/1  "Beta"
  Constant8/1 -> Sum6/2
  Sum6/1 -> Relational Operator1/2
  Sum2/1 -> Sum4/2
  Sum4/1 -> Math Function/1
  Logical Operator/1 -> Logical Operator2/1, Mux3/1
  Logical Operator2/1 -> Mux3/2
  Mux3/1 -> Selector3/1
  Selector3/1 -> Pulses/1
  Gain3/1 -> Sum6/1
  Math Function/1 -> Relational Operator1/1, Relational Operator/1
  wt/1 -> Sum2/1  "wt"
  Constant2/1 -> Math Function/2

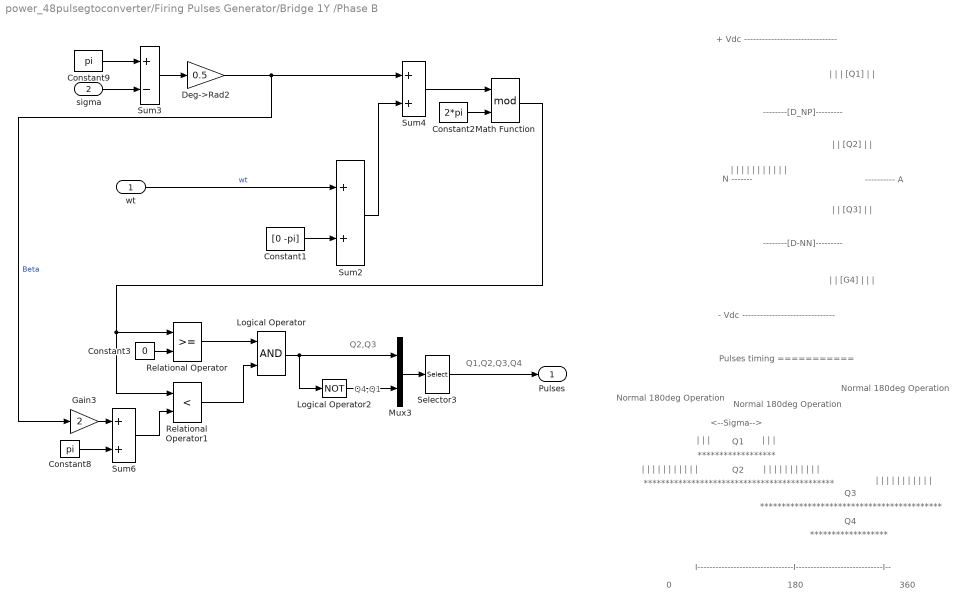
== system power_48pulsegtoconverter/Firing Pulses Generator/Bridge 1Y /Phase B ==
  note: <--Sigma-->
  note: |
      | |
      | |
  note: |
      | |
      | |
  note: Q4
  note: Q3
  note: Q2
  note: Q1
  note: ******************************************
  note: ********************************************
  note: ******************
  note: ******************
  note: 360
  note: 180
  note: 0
  note: I--------------------------------I-----------------------------I--
  note: Normal 180deg
      | Operation
  note: Normal 180deg
      | Operation
  note: Normal 180deg
      | Operation
  note: Pulses timing
      | ===========
  note: |
      | |
      | |
      | |
      | |
      | |
      | |
      | |
      | |
      | |
      | |
  note: |
      | |
      | |
      | |
      | |
      | |
      | |
      | |
      | |
      | |
      | |
  note: |
      | |
      | |
      | |
      | |
      | |
      | |
      | |
      | |
      | |
      | |
  note: Q1,Q2,Q3,Q4
  note: Q2,Q3
  note: Q4,Q1
  note: + Vdc -------------------------------
  note: - Vdc -------------------------------
  note: N -------
  note: |
      | |
      | |
      | |
      | |
      | |
      | |
      | |
      | |
      | |
      | |
  note: ---------- A
  note: --------[D-NN]---------
  note: --------[D_NP]---------
  note: |
      | |
      | [G4]
      | |
      | |
      | |
  note: |
      | |
      | [Q3]
      | |
      | |
  note: |
      | |
      | [Q2]
      | |
      | |
  note: |
      | |
      | |
      | [Q1]
      | |
      | |
  wt : Inport  PortDimensions=1
  sigma : Inport  Port=2  PortDimensions=1
  Constant1 : Constant  Value=[0 -pi]
  Constant2 : Constant  Value=2*pi
  Constant3 : Constant  Value=0
  Constant8 : Constant  Value=pi
  Constant9 : Constant  Value=pi
  Deg->Rad2 : Gain  Gain=0.5  SaturateOnIntegerOverflow=on  OutDataTypeStr=Inherit: Same as input  ParamDataTypeStr=Inherit: Same as input
  Gain3 : Gain  Gain=2  SaturateOnIntegerOverflow=on  OutDataTypeStr=Inherit: Same as input  ParamDataTypeStr=Inherit: Same as input
  Logical Operator : Logic
  Logical Operator2 : Logic  Operator=NOT
  Math Function : Math  Operator=mod  SaturateOnIntegerOverflow=on
  Mux3 : Mux  Inputs=[2 2]
  Relational Operator : RelationalOperator  ZeroCross=off  InputSameDT=on
  Relational Operator1 : RelationalOperator  Operator=<  ZeroCross=off  InputSameDT=on
  Selector3 : Selector  InputPortWidth=4  IndexOptions=Index vector (dialog)  Indices=[4 1 2 3]  OutputSizes=1
  Sum2 : Sum  SaturateOnIntegerOverflow=on  InputSameDT=on  OutDataTypeStr=Inherit: Same as first input
  Sum3 : Sum  Inputs=+-  SaturateOnIntegerOverflow=on  InputSameDT=on  OutDataTypeStr=Inherit: Same as first input
  Sum4 : Sum  SaturateOnIntegerOverflow=on  InputSameDT=on  OutDataTypeStr=Inherit: Same as first input
  Sum6 : Sum  SaturateOnIntegerOverflow=on  InputSameDT=on  OutDataTypeStr=Inherit: Same as first input
  Pulses : Outport
  wires:
  Constant2/1 -> Math Function/2
  wt/1 -> Sum2/1  "wt"
  Math Function/1 -> Relational Operator/1, Relational Operator1/1
  Gain3/1 -> Sum6/1
  Selector3/1 -> Pulses/1
  Mux3/1 -> Selector3/1
  Logical Operator2/1 -> Mux3/2
  Logical Operator/1 -> Mux3/1, Logical Operator2/1
  Sum4/1 -> Math Function/1
  Sum2/1 -> Sum4/2
  Sum6/1 -> Relational Operator1/2
  Constant8/1 -> Sum6/2
  Deg->Rad2/1 -> Gain3/1, Sum4/1  "Beta"
  Sum3/1 -> Deg->Rad2/1
  sigma/1 -> Sum3/2
  Constant9/1 -> Sum3/1
  Relational Operator1/1 -> Logical Operator/2
  Relational Operator/1 -> Logical Operator/1
  Constant3/1 -> Relational Operator/2
  Constant1/1 -> Sum2/2

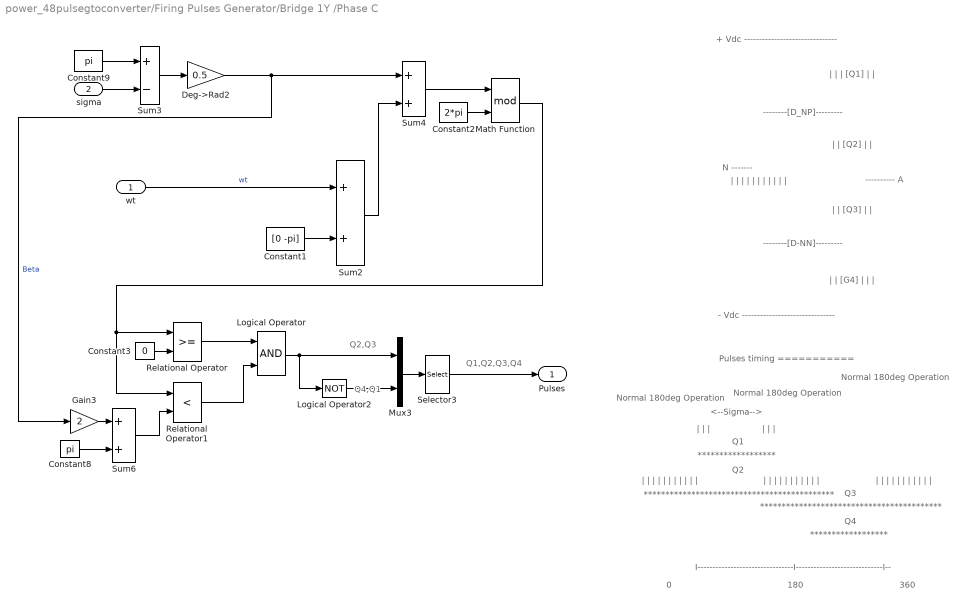
== system power_48pulsegtoconverter/Firing Pulses Generator/Bridge 1Y /Phase C ==
  note: |
      | |
      | |
      | [Q1]
      | |
      | |
  note: |
      | |
      | [Q2]
      | |
      | |
  note: |
      | |
      | [Q3]
      | |
      | |
  note: |
      | |
      | [G4]
      | |
      | |
      | |
  note: --------[D_NP]---------
  note: --------[D-NN]---------
  note: ---------- A
  note: |
      | |
      | |
      | |
      | |
      | |
      | |
      | |
      | |
      | |
      | |
  note: N -------
  note: - Vdc -------------------------------
  note: + Vdc -------------------------------
  note: Q4,Q1
  note: Q2,Q3
  note: Q1,Q2,Q3,Q4
  note: |
      | |
      | |
      | |
      | |
      | |
      | |
      | |
      | |
      | |
      | |
  note: |
      | |
      | |
      | |
      | |
      | |
      | |
      | |
      | |
      | |
      | |
  note: |
      | |
      | |
      | |
      | |
      | |
      | |
      | |
      | |
      | |
      | |
  note: Pulses timing
      | ===========
  note: Normal 180deg
      | Operation
  note: Normal 180deg
      | Operation
  note: Normal 180deg
      | Operation
  note: I--------------------------------I-----------------------------I--
  note: 0
  note: 180
  note: 360
  note: ******************
  note: ******************
  note: ********************************************
  note: ******************************************
  note: Q1
  note: Q2
  note: Q3
  note: Q4
  note: |
      | |
      | |
  note: |
      | |
      | |
  note: <--Sigma-->
  wt : Inport  PortDimensions=1
  sigma : Inport  Port=2  PortDimensions=1
  Constant1 : Constant  Value=[0 -pi]
  Constant2 : Constant  Value=2*pi
  Constant3 : Constant  Value=0
  Constant8 : Constant  Value=pi
  Constant9 : Constant  Value=pi
  Deg->Rad2 : Gain  Gain=0.5  SaturateOnIntegerOverflow=on  OutDataTypeStr=Inherit: Same as input  ParamDataTypeStr=Inherit: Same as input
  Gain3 : Gain  Gain=2  SaturateOnIntegerOverflow=on  OutDataTypeStr=Inherit: Same as input  ParamDataTypeStr=Inherit: Same as input
  Logical Operator : Logic
  Logical Operator2 : Logic  Operator=NOT
  Math Function : Math  Operator=mod  SaturateOnIntegerOverflow=on
  Mux3 : Mux  Inputs=[2 2]
  Relational Operator : RelationalOperator  ZeroCross=off  InputSameDT=on
  Relational Operator1 : RelationalOperator  Operator=<  ZeroCross=off  InputSameDT=on
  Selector3 : Selector  InputPortWidth=4  IndexOptions=Index vector (dialog)  Indices=[4 1 2 3]  OutputSizes=1
  Sum2 : Sum  SaturateOnIntegerOverflow=on  InputSameDT=on  OutDataTypeStr=Inherit: Same as first input
  Sum3 : Sum  Inputs=+-  SaturateOnIntegerOverflow=on  InputSameDT=on  OutDataTypeStr=Inherit: Same as first input
  Sum4 : Sum  SaturateOnIntegerOverflow=on  InputSameDT=on  OutDataTypeStr=Inherit: Same as first input
  Sum6 : Sum  SaturateOnIntegerOverflow=on  InputSameDT=on  OutDataTypeStr=Inherit: Same as first input
  Pulses : Outport
  wires:
  Constant1/1 -> Sum2/2
  Constant3/1 -> Relational Operator/2
  Relational Operator/1 -> Logical Operator/1
  Relational Operator1/1 -> Logical Operator/2
  Constant9/1 -> Sum3/1
  sigma/1 -> Sum3/2
  Sum3/1 -> Deg->Rad2/1
  Deg->Rad2/1 -> Sum4/1, Gain3/1  "Beta"
  Constant8/1 -> Sum6/2
  Sum6/1 -> Relational Operator1/2
  Sum2/1 -> Sum4/2
  Sum4/1 -> Math Function/1
  Logical Operator/1 -> Logical Operator2/1, Mux3/1
  Logical Operator2/1 -> Mux3/2
  Mux3/1 -> Selector3/1
  Selector3/1 -> Pulses/1
  Gain3/1 -> Sum6/1
  Math Function/1 -> Relational Operator1/1, Relational Operator/1
  wt/1 -> Sum2/1  "wt"
  Constant2/1 -> Math Function/2

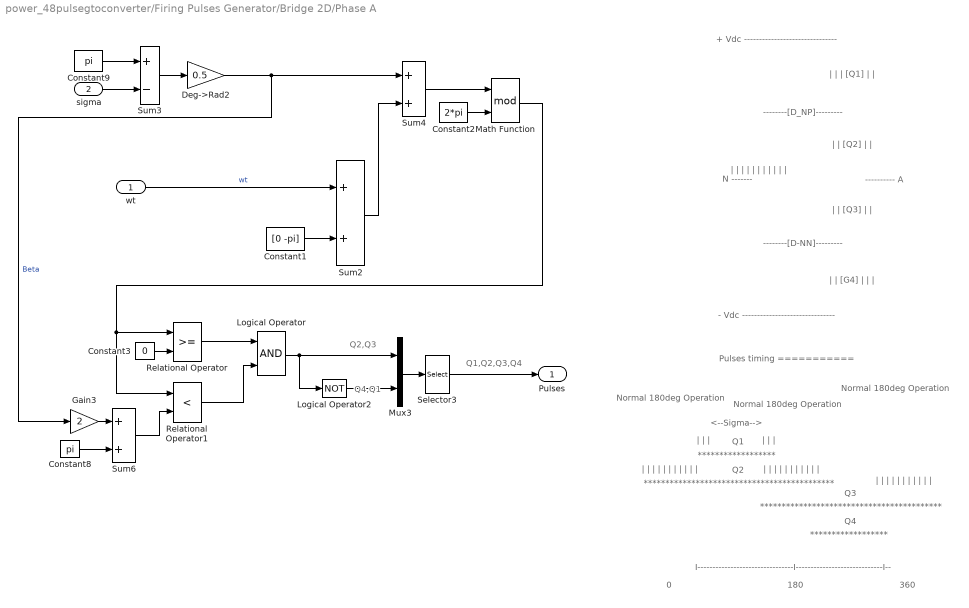
== system power_48pulsegtoconverter/Firing Pulses Generator/Bridge 2D/Phase A ==
  note: <--Sigma-->
  note: |
      | |
      | |
  note: |
      | |
      | |
  note: Q4
  note: Q3
  note: Q2
  note: Q1
  note: ******************************************
  note: ********************************************
  note: ******************
  note: ******************
  note: 360
  note: 180
  note: 0
  note: I--------------------------------I-----------------------------I--
  note: Normal 180deg
      | Operation
  note: Normal 180deg
      | Operation
  note: Normal 180deg
      | Operation
  note: Pulses timing
      | ===========
  note: |
      | |
      | |
      | |
      | |
      | |
      | |
      | |
      | |
      | |
      | |
  note: |
      | |
      | |
      | |
      | |
      | |
      | |
      | |
      | |
      | |
      | |
  note: |
      | |
      | |
      | |
      | |
      | |
      | |
      | |
      | |
      | |
      | |
  note: Q1,Q2,Q3,Q4
  note: Q2,Q3
  note: Q4,Q1
  note: + Vdc -------------------------------
  note: - Vdc -------------------------------
  note: N -------
  note: |
      | |
      | |
      | |
      | |
      | |
      | |
      | |
      | |
      | |
      | |
  note: ---------- A
  note: --------[D-NN]---------
  note: --------[D_NP]---------
  note: |
      | |
      | [G4]
      | |
      | |
      | |
  note: |
      | |
      | [Q3]
      | |
      | |
  note: |
      | |
      | [Q2]
      | |
      | |
  note: |
      | |
      | |
      | [Q1]
      | |
      | |
  wt : Inport  PortDimensions=1
  sigma : Inport  Port=2  PortDimensions=1
  Constant1 : Constant  Value=[0 -pi]
  Constant2 : Constant  Value=2*pi
  Constant3 : Constant  Value=0
  Constant8 : Constant  Value=pi
  Constant9 : Constant  Value=pi
  Deg->Rad2 : Gain  Gain=0.5  SaturateOnIntegerOverflow=on  OutDataTypeStr=Inherit: Same as input  ParamDataTypeStr=Inherit: Same as input
  Gain3 : Gain  Gain=2  SaturateOnIntegerOverflow=on  OutDataTypeStr=Inherit: Same as input  ParamDataTypeStr=Inherit: Same as input
  Logical Operator : Logic
  Logical Operator2 : Logic  Operator=NOT
  Math Function : Math  Operator=mod  SaturateOnIntegerOverflow=on
  Mux3 : Mux  Inputs=[2 2]
  Relational Operator : RelationalOperator  ZeroCross=off  InputSameDT=on
  Relational Operator1 : RelationalOperator  Operator=<  ZeroCross=off  InputSameDT=on
  Selector3 : Selector  InputPortWidth=4  IndexOptions=Index vector (dialog)  Indices=[4 1 2 3]  OutputSizes=1
  Sum2 : Sum  SaturateOnIntegerOverflow=on  InputSameDT=on  OutDataTypeStr=Inherit: Same as first input
  Sum3 : Sum  Inputs=+-  SaturateOnIntegerOverflow=on  InputSameDT=on  OutDataTypeStr=Inherit: Same as first input
  Sum4 : Sum  SaturateOnIntegerOverflow=on  InputSameDT=on  OutDataTypeStr=Inherit: Same as first input
  Sum6 : Sum  SaturateOnIntegerOverflow=on  InputSameDT=on  OutDataTypeStr=Inherit: Same as first input
  Pulses : Outport
  wires:
  Constant2/1 -> Math Function/2
  wt/1 -> Sum2/1  "wt"
  Math Function/1 -> Relational Operator/1, Relational Operator1/1
  Gain3/1 -> Sum6/1
  Selector3/1 -> Pulses/1
  Mux3/1 -> Selector3/1
  Logical Operator2/1 -> Mux3/2
  Logical Operator/1 -> Mux3/1, Logical Operator2/1
  Sum4/1 -> Math Function/1
  Sum2/1 -> Sum4/2
  Sum6/1 -> Relational Operator1/2
  Constant8/1 -> Sum6/2
  Deg->Rad2/1 -> Gain3/1, Sum4/1  "Beta"
  Sum3/1 -> Deg->Rad2/1
  sigma/1 -> Sum3/2
  Constant9/1 -> Sum3/1
  Relational Operator1/1 -> Logical Operator/2
  Relational Operator/1 -> Logical Operator/1
  Constant3/1 -> Relational Operator/2
  Constant1/1 -> Sum2/2

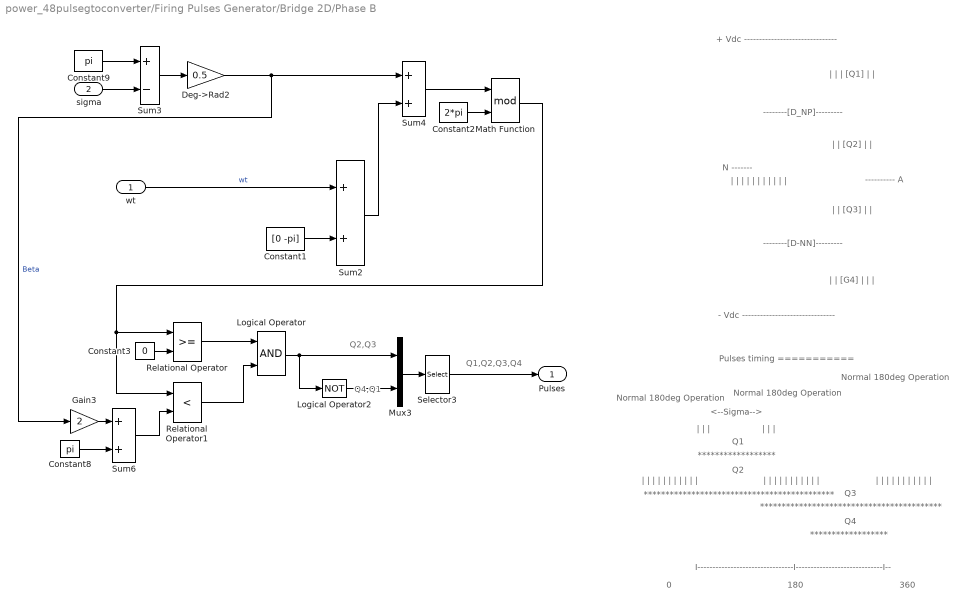
== system power_48pulsegtoconverter/Firing Pulses Generator/Bridge 2D/Phase B ==
  note: |
      | |
      | |
      | [Q1]
      | |
      | |
  note: |
      | |
      | [Q2]
      | |
      | |
  note: |
      | |
      | [Q3]
      | |
      | |
  note: |
      | |
      | [G4]
      | |
      | |
      | |
  note: --------[D_NP]---------
  note: --------[D-NN]---------
  note: ---------- A
  note: |
      | |
      | |
      | |
      | |
      | |
      | |
      | |
      | |
      | |
      | |
  note: N -------
  note: - Vdc -------------------------------
  note: + Vdc -------------------------------
  note: Q4,Q1
  note: Q2,Q3
  note: Q1,Q2,Q3,Q4
  note: |
      | |
      | |
      | |
      | |
      | |
      | |
      | |
      | |
      | |
      | |
  note: |
      | |
      | |
      | |
      | |
      | |
      | |
      | |
      | |
      | |
      | |
  note: |
      | |
      | |
      | |
      | |
      | |
      | |
      | |
      | |
      | |
      | |
  note: Pulses timing
      | ===========
  note: Normal 180deg
      | Operation
  note: Normal 180deg
      | Operation
  note: Normal 180deg
      | Operation
  note: I--------------------------------I-----------------------------I--
  note: 0
  note: 180
  note: 360
  note: ******************
  note: ******************
  note: ********************************************
  note: ******************************************
  note: Q1
  note: Q2
  note: Q3
  note: Q4
  note: |
      | |
      | |
  note: |
      | |
      | |
  note: <--Sigma-->
  wt : Inport  PortDimensions=1
  sigma : Inport  Port=2  PortDimensions=1
  Constant1 : Constant  Value=[0 -pi]
  Constant2 : Constant  Value=2*pi
  Constant3 : Constant  Value=0
  Constant8 : Constant  Value=pi
  Constant9 : Constant  Value=pi
  Deg->Rad2 : Gain  Gain=0.5  SaturateOnIntegerOverflow=on  OutDataTypeStr=Inherit: Same as input  ParamDataTypeStr=Inherit: Same as input
  Gain3 : Gain  Gain=2  SaturateOnIntegerOverflow=on  OutDataTypeStr=Inherit: Same as input  ParamDataTypeStr=Inherit: Same as input
  Logical Operator : Logic
  Logical Operator2 : Logic  Operator=NOT
  Math Function : Math  Operator=mod  SaturateOnIntegerOverflow=on
  Mux3 : Mux  Inputs=[2 2]
  Relational Operator : RelationalOperator  ZeroCross=off  InputSameDT=on
  Relational Operator1 : RelationalOperator  Operator=<  ZeroCross=off  InputSameDT=on
  Selector3 : Selector  InputPortWidth=4  IndexOptions=Index vector (dialog)  Indices=[4 1 2 3]  OutputSizes=1
  Sum2 : Sum  SaturateOnIntegerOverflow=on  InputSameDT=on  OutDataTypeStr=Inherit: Same as first input
  Sum3 : Sum  Inputs=+-  SaturateOnIntegerOverflow=on  InputSameDT=on  OutDataTypeStr=Inherit: Same as first input
  Sum4 : Sum  SaturateOnIntegerOverflow=on  InputSameDT=on  OutDataTypeStr=Inherit: Same as first input
  Sum6 : Sum  SaturateOnIntegerOverflow=on  InputSameDT=on  OutDataTypeStr=Inherit: Same as first input
  Pulses : Outport
  wires:
  Constant1/1 -> Sum2/2
  Constant3/1 -> Relational Operator/2
  Relational Operator/1 -> Logical Operator/1
  Relational Operator1/1 -> Logical Operator/2
  Constant9/1 -> Sum3/1
  sigma/1 -> Sum3/2
  Sum3/1 -> Deg->Rad2/1
  Deg->Rad2/1 -> Sum4/1, Gain3/1  "Beta"
  Constant8/1 -> Sum6/2
  Sum6/1 -> Relational Operator1/2
  Sum2/1 -> Sum4/2
  Sum4/1 -> Math Function/1
  Logical Operator/1 -> Logical Operator2/1, Mux3/1
  Logical Operator2/1 -> Mux3/2
  Mux3/1 -> Selector3/1
  Selector3/1 -> Pulses/1
  Gain3/1 -> Sum6/1
  Math Function/1 -> Relational Operator1/1, Relational Operator/1
  wt/1 -> Sum2/1  "wt"
  Constant2/1 -> Math Function/2

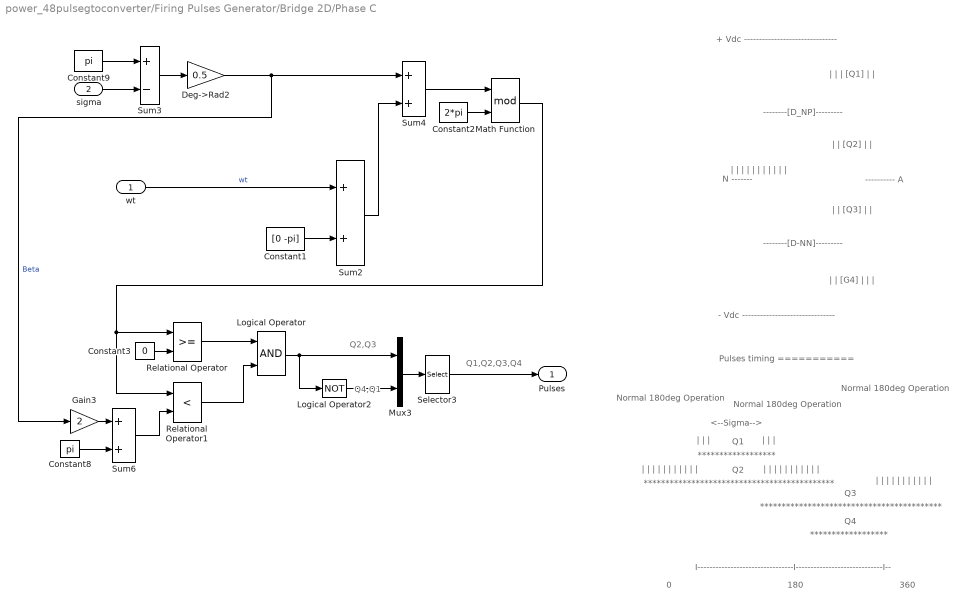
== system power_48pulsegtoconverter/Firing Pulses Generator/Bridge 2D/Phase C ==
  note: <--Sigma-->
  note: |
      | |
      | |
  note: |
      | |
      | |
  note: Q4
  note: Q3
  note: Q2
  note: Q1
  note: ******************************************
  note: ********************************************
  note: ******************
  note: ******************
  note: 360
  note: 180
  note: 0
  note: I--------------------------------I-----------------------------I--
  note: Normal 180deg
      | Operation
  note: Normal 180deg
      | Operation
  note: Normal 180deg
      | Operation
  note: Pulses timing
      | ===========
  note: |
      | |
      | |
      | |
      | |
      | |
      | |
      | |
      | |
      | |
      | |
  note: |
      | |
      | |
      | |
      | |
      | |
      | |
      | |
      | |
      | |
      | |
  note: |
      | |
      | |
      | |
      | |
      | |
      | |
      | |
      | |
      | |
      | |
  note: Q1,Q2,Q3,Q4
  note: Q2,Q3
  note: Q4,Q1
  note: + Vdc -------------------------------
  note: - Vdc -------------------------------
  note: N -------
  note: |
      | |
      | |
      | |
      | |
      | |
      | |
      | |
      | |
      | |
      | |
  note: ---------- A
  note: --------[D-NN]---------
  note: --------[D_NP]---------
  note: |
      | |
      | [G4]
      | |
      | |
      | |
  note: |
      | |
      | [Q3]
      | |
      | |
  note: |
      | |
      | [Q2]
      | |
      | |
  note: |
      | |
      | |
      | [Q1]
      | |
      | |
  wt : Inport  PortDimensions=1
  sigma : Inport  Port=2  PortDimensions=1
  Constant1 : Constant  Value=[0 -pi]
  Constant2 : Constant  Value=2*pi
  Constant3 : Constant  Value=0
  Constant8 : Constant  Value=pi
  Constant9 : Constant  Value=pi
  Deg->Rad2 : Gain  Gain=0.5  SaturateOnIntegerOverflow=on  OutDataTypeStr=Inherit: Same as input  ParamDataTypeStr=Inherit: Same as input
  Gain3 : Gain  Gain=2  SaturateOnIntegerOverflow=on  OutDataTypeStr=Inherit: Same as input  ParamDataTypeStr=Inherit: Same as input
  Logical Operator : Logic
  Logical Operator2 : Logic  Operator=NOT
  Math Function : Math  Operator=mod  SaturateOnIntegerOverflow=on
  Mux3 : Mux  Inputs=[2 2]
  Relational Operator : RelationalOperator  ZeroCross=off  InputSameDT=on
  Relational Operator1 : RelationalOperator  Operator=<  ZeroCross=off  InputSameDT=on
  Selector3 : Selector  InputPortWidth=4  IndexOptions=Index vector (dialog)  Indices=[4 1 2 3]  OutputSizes=1
  Sum2 : Sum  SaturateOnIntegerOverflow=on  InputSameDT=on  OutDataTypeStr=Inherit: Same as first input
  Sum3 : Sum  Inputs=+-  SaturateOnIntegerOverflow=on  InputSameDT=on  OutDataTypeStr=Inherit: Same as first input
  Sum4 : Sum  SaturateOnIntegerOverflow=on  InputSameDT=on  OutDataTypeStr=Inherit: Same as first input
  Sum6 : Sum  SaturateOnIntegerOverflow=on  InputSameDT=on  OutDataTypeStr=Inherit: Same as first input
  Pulses : Outport
  wires:
  Constant2/1 -> Math Function/2
  wt/1 -> Sum2/1  "wt"
  Math Function/1 -> Relational Operator/1, Relational Operator1/1
  Gain3/1 -> Sum6/1
  Selector3/1 -> Pulses/1
  Mux3/1 -> Selector3/1
  Logical Operator2/1 -> Mux3/2
  Logical Operator/1 -> Mux3/1, Logical Operator2/1
  Sum4/1 -> Math Function/1
  Sum2/1 -> Sum4/2
  Sum6/1 -> Relational Operator1/2
  Constant8/1 -> Sum6/2
  Deg->Rad2/1 -> Gain3/1, Sum4/1  "Beta"
  Sum3/1 -> Deg->Rad2/1
  sigma/1 -> Sum3/2
  Constant9/1 -> Sum3/1
  Relational Operator1/1 -> Logical Operator/2
  Relational Operator/1 -> Logical Operator/1
  Constant3/1 -> Relational Operator/2
  Constant1/1 -> Sum2/2

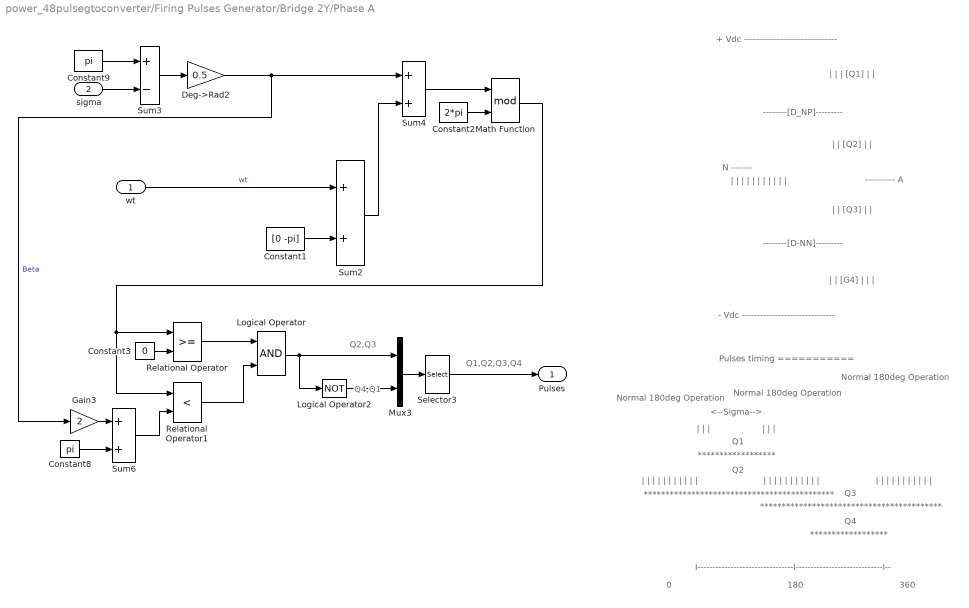
== system power_48pulsegtoconverter/Firing Pulses Generator/Bridge 2Y/Phase A ==
  note: |
      | |
      | |
      | [Q1]
      | |
      | |
  note: |
      | |
      | [Q2]
      | |
      | |
  note: |
      | |
      | [Q3]
      | |
      | |
  note: |
      | |
      | [G4]
      | |
      | |
      | |
  note: --------[D_NP]---------
  note: --------[D-NN]---------
  note: ---------- A
  note: |
      | |
      | |
      | |
      | |
      | |
      | |
      | |
      | |
      | |
      | |
  note: N -------
  note: - Vdc -------------------------------
  note: + Vdc -------------------------------
  note: Q4,Q1
  note: Q2,Q3
  note: Q1,Q2,Q3,Q4
  note: |
      | |
      | |
      | |
      | |
      | |
      | |
      | |
      | |
      | |
      | |
  note: |
      | |
      | |
      | |
      | |
      | |
      | |
      | |
      | |
      | |
      | |
  note: |
      | |
      | |
      | |
      | |
      | |
      | |
      | |
      | |
      | |
      | |
  note: Pulses timing
      | ===========
  note: Normal 180deg
      | Operation
  note: Normal 180deg
      | Operation
  note: Normal 180deg
      | Operation
  note: I--------------------------------I-----------------------------I--
  note: 0
  note: 180
  note: 360
  note: ******************
  note: ******************
  note: ********************************************
  note: ******************************************
  note: Q1
  note: Q2
  note: Q3
  note: Q4
  note: |
      | |
      | |
  note: |
      | |
      | |
  note: <--Sigma-->
  wt : Inport  PortDimensions=1
  sigma : Inport  Port=2  PortDimensions=1
  Constant1 : Constant  Value=[0 -pi]
  Constant2 : Constant  Value=2*pi
  Constant3 : Constant  Value=0
  Constant8 : Constant  Value=pi
  Constant9 : Constant  Value=pi
  Deg->Rad2 : Gain  Gain=0.5  SaturateOnIntegerOverflow=on  OutDataTypeStr=Inherit: Same as input  ParamDataTypeStr=Inherit: Same as input
  Gain3 : Gain  Gain=2  SaturateOnIntegerOverflow=on  OutDataTypeStr=Inherit: Same as input  ParamDataTypeStr=Inherit: Same as input
  Logical Operator : Logic
  Logical Operator2 : Logic  Operator=NOT
  Math Function : Math  Operator=mod  SaturateOnIntegerOverflow=on
  Mux3 : Mux  Inputs=[2 2]
  Relational Operator : RelationalOperator  ZeroCross=off  InputSameDT=on
  Relational Operator1 : RelationalOperator  Operator=<  ZeroCross=off  InputSameDT=on
  Selector3 : Selector  InputPortWidth=4  IndexOptions=Index vector (dialog)  Indices=[4 1 2 3]  OutputSizes=1
  Sum2 : Sum  SaturateOnIntegerOverflow=on  InputSameDT=on  OutDataTypeStr=Inherit: Same as first input
  Sum3 : Sum  Inputs=+-  SaturateOnIntegerOverflow=on  InputSameDT=on  OutDataTypeStr=Inherit: Same as first input
  Sum4 : Sum  SaturateOnIntegerOverflow=on  InputSameDT=on  OutDataTypeStr=Inherit: Same as first input
  Sum6 : Sum  SaturateOnIntegerOverflow=on  InputSameDT=on  OutDataTypeStr=Inherit: Same as first input
  Pulses : Outport
  wires:
  Constant1/1 -> Sum2/2
  Constant3/1 -> Relational Operator/2
  Relational Operator/1 -> Logical Operator/1
  Relational Operator1/1 -> Logical Operator/2
  Constant9/1 -> Sum3/1
  sigma/1 -> Sum3/2
  Sum3/1 -> Deg->Rad2/1
  Deg->Rad2/1 -> Sum4/1, Gain3/1  "Beta"
  Constant8/1 -> Sum6/2
  Sum6/1 -> Relational Operator1/2
  Sum2/1 -> Sum4/2
  Sum4/1 -> Math Function/1
  Logical Operator/1 -> Logical Operator2/1, Mux3/1
  Logical Operator2/1 -> Mux3/2
  Mux3/1 -> Selector3/1
  Selector3/1 -> Pulses/1
  Gain3/1 -> Sum6/1
  Math Function/1 -> Relational Operator1/1, Relational Operator/1
  wt/1 -> Sum2/1  "wt"
  Constant2/1 -> Math Function/2
